simulink model "sgMdl_IO623_FlexRayLoopback"  (R2024b)
settings: Solver=FixedStepAuto  StartTime=0.0  StopTime=inf  RelTol=1e-3  EnableMultiTasking=on
undefined symbols (not defined in the file): IO623
libraries: speedgoatlib_IO623 x8, speedgoatlib_interrupt x1
Description:
  | IO623 - Loopback Test
settings Model: ModifiedByFormat=Speedgoat  SimulationMode=external  Creator=Speedgoat  LastModifiedBy=Speedgoat
settings SolverCC: ConcurrentTasks=on  AlgebraicLoopSolver=TrustRegion  PositivePriorityOrder=on  AutoInsertRateTranBlk=on
settings DataIOCC: SaveFormat=StructureWithTime
settings OptimizationCC: BlockReduction=off  OptimizeBlockIOStorage=off  ReuseModelBlockBuffer=off
settings DebuggingCC: TasksWithSamePriorityMsg=none  UnconnectedInputMsg=warning  UnconnectedOutputMsg=warning  UnconnectedLineMsg=warning
settings HardwareCC: ProdBitPerLong=64  ProdLongLongMode=on  ProdHWDeviceType=Intel->x86-64 (Linux 64)
settings ModelReferenceCC: EnableRefExpFcnMdlSchedulingChecks=on
settings RTWCC: Description=Speedgoat Real-Time Target Machine  SystemTargetFile=speedgoat.tlc  TemplateMakefile=slrealtime_default_tmf  PostCodeGenCommand=sg.model.build.makeCfg(bdroot, buildInfo);  Toolchain=Simulink Real-Time Toolchain  BuildConfiguration=Faster Runs  TargetLang=C++  GPUComputeCapability=3.5  DLArmComputeVersion=19.05
settings SimulinkRealTimeTargetCC: SubcomponentCodeInterfacePackaging=Reusable function  InstructionSetFMA=off  LogToMDFFile=off  SLRTFileLogMaxRuns=10  UseGCCFastMath=on
settings ConfigComp: CovBoundaryAbsTol=1.0e-5

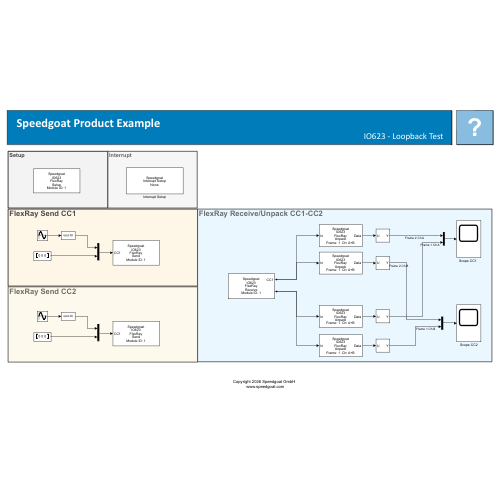
[thumbnail: Simulink's stored preview of the top-level diagram]
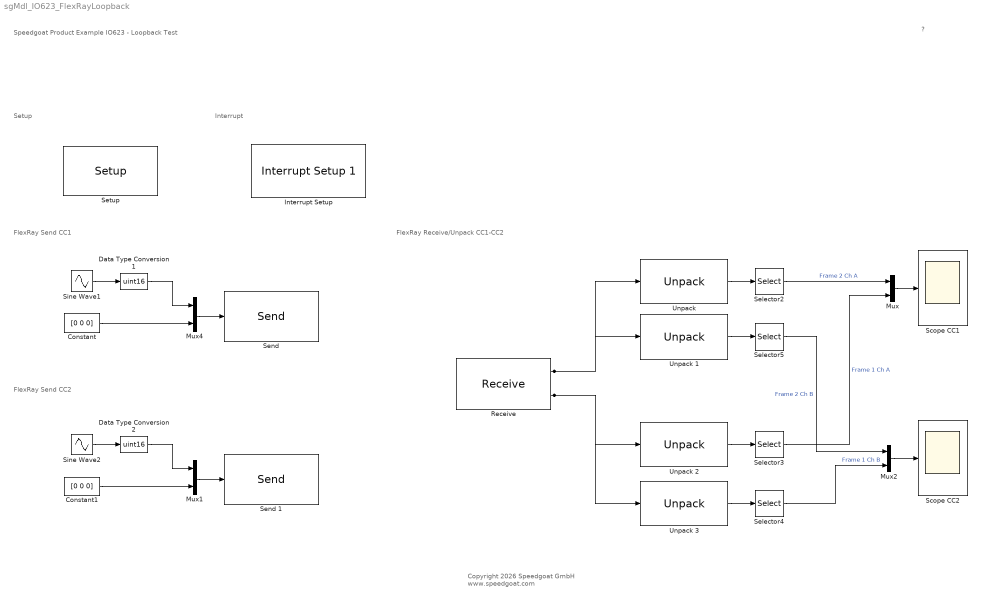
== system sgMdl_IO623_FlexRayLoopback ==
  note: FlexRay Receive/Unpack CC1-CC2
  note: FlexRay Send CC1
  note: FlexRay Send CC2
  note: Interrupt
  note: Setup
  note: Speedgoat Product Example
      | IO623 - Loopback Test
  note: ?
  note: Copyright 2026 Speedgoat GmbH
      |  www.speedgoat.com
  Constant : Constant  Value=[0 0 0]  OutDataTypeStr=uint16
  Constant1 : Constant  Value=[0 0 0]  OutDataTypeStr=uint16
  Data Type Conversion1 : DataTypeConversion  OutDataTypeStr=uint16  SaturateOnIntegerOverflow=off  RndMeth=Floor
  Data Type Conversion2 : DataTypeConversion  OutDataTypeStr=uint16  SaturateOnIntegerOverflow=off  RndMeth=Floor
  Interrupt Setup : speedgoatlib_interrupt/Interrupt Setup 1  parModuleTrigger=on  parPollingMode=off  parPriorityConf=High  parPriority=254  confStartFcn=IO623_start_public  confStopFcn=IO623_stop_public  confIsrFcn=IO623_isr_public  confMapFcn=IO623_map_public  confHookFile=io623_int_hooks.cpp  confIrqNr=-1  confIsPolling=off  confModID=16776961  confSelectedInt=Speedgoat IO623 interrupt  confSelectedId=1  confSelectedChannel=[]  confData=[]  confForcePollingMode=off
  Mux{,1..2,4} (4 alike) : Mux  Inputs=2
  "Receive " : speedgoatlib_IO623/Receive   parModuleId=1  parMaxFrames=10  parSampleTime=-1  parPciSlot=-1  parActiveControllers=[1 1 0 0]
      settings: SourceProductName=Simulink Real-Time: Speedgoat I/O Blockset
  "Scope CC1  " : Scope
  Scope CC2 : Scope
  Selector{2..5} (4 alike) : Selector  InputPortWidth=127  IndexOptions=Index vector (dialog)  Indices=1  OutputSizes=1
  "Send " : speedgoatlib_IO623/Send   parModuleId=1  parCommController=CC1  parSelectionInfo=Frame ID: 1, Channel: A+B, Base: 0, Rep.: 1  parPayloadLength=-1  parSampleTime=-1  parPciSlot=-1  parActiveControllers=[1 1 0 0]
      settings: SourceProductName=Simulink Real-Time: Speedgoat I/O Blockset
  Send 1 : speedgoatlib_IO623/Send   parModuleId=1  parCommController=CC2  parSelectionInfo=Frame ID: 2, Channel: A+B, Base: 0, Rep.: 1  parPayloadLength=-1  parSampleTime=-1  parPciSlot=-1  parActiveControllers=[1 1 0 0]
      settings: SourceProductName=Simulink Real-Time: Speedgoat I/O Blockset
  "Setup " : speedgoatlib_IO623/Setup   parModuleId=1  parPciSlot=-1  parModuleVariant=IO623-2  parChiFile1=config_cc1.chi  parEnableCc1=on  parBusTermination1=on  parChiFile2=config_cc2.chi  parEnableCc2=on  parBusTermination2=off  parEnableCc3=on  parBusTermination3=off  parEnableCc4=on  parBusTermination4=off
      settings: SourceProductName=Simulink Real-Time: Speedgoat I/O Blockset
  Sine Wave1 : Sin  Amplitude=32767  Bias=32768  Frequency=5*2*pi
  Sine Wave2 : Sin  Amplitude=32767  Bias=32768  Frequency=5*2*pi  Phase=2*pi*1/4
  "Unpack " : speedgoatlib_IO623/Unpack   parFrameId=2  parChannels=A  parIgnoreNullFrames=on  parEnPortPayloadPreambleInd=off  parEnPortNullFrameInd=off  parEnPortSyncFrameInd=off  parEnPortStartupFrameInd=off  parEnPortPayloadLength=off  parEnPortHeaderCrc=off  parEnPortCycleCount=off  parEnPortData=on  parEnPortChannel=off  parEnPortValidFrame=off  parEnPortSyntaxError=off  parEnPortContentError=off  parEnPortSlotBoundaryViolation=off  parEnPortTimestamp=off
      settings: SourceProductName=Simulink Real-Time: Speedgoat I/O Blockset
  Unpack 1 : speedgoatlib_IO623/Unpack   parFrameId=2  parChannels=B  parIgnoreNullFrames=on  parEnPortPayloadPreambleInd=off  parEnPortNullFrameInd=off  parEnPortSyncFrameInd=off  parEnPortStartupFrameInd=off  parEnPortPayloadLength=off  parEnPortHeaderCrc=off  parEnPortCycleCount=off  parEnPortData=on  parEnPortChannel=off  parEnPortValidFrame=off  parEnPortSyntaxError=off  parEnPortContentError=off  parEnPortSlotBoundaryViolation=off  parEnPortTimestamp=off
      settings: SourceProductName=Simulink Real-Time: Speedgoat I/O Blockset
  Unpack 2 : speedgoatlib_IO623/Unpack   parFrameId=1  parChannels=A  parIgnoreNullFrames=on  parEnPortPayloadPreambleInd=off  parEnPortNullFrameInd=off  parEnPortSyncFrameInd=off  parEnPortStartupFrameInd=off  parEnPortPayloadLength=off  parEnPortHeaderCrc=off  parEnPortCycleCount=off  parEnPortData=on  parEnPortChannel=off  parEnPortValidFrame=off  parEnPortSyntaxError=off  parEnPortContentError=off  parEnPortSlotBoundaryViolation=off  parEnPortTimestamp=off
      settings: SourceProductName=Simulink Real-Time: Speedgoat I/O Blockset
  Unpack 3 : speedgoatlib_IO623/Unpack   parFrameId=1  parChannels=B  parIgnoreNullFrames=on  parEnPortPayloadPreambleInd=off  parEnPortNullFrameInd=off  parEnPortSyncFrameInd=off  parEnPortStartupFrameInd=off  parEnPortPayloadLength=off  parEnPortHeaderCrc=off  parEnPortCycleCount=off  parEnPortData=on  parEnPortChannel=off  parEnPortValidFrame=off  parEnPortSyntaxError=off  parEnPortContentError=off  parEnPortSlotBoundaryViolation=off  parEnPortTimestamp=off
      settings: SourceProductName=Simulink Real-Time: Speedgoat I/O Blockset
  wires:
  Mux1/1 -> Send 1/1
  Constant1/1 -> Mux1/2
  Selector5/1 -> Mux2/1  "Frame 2 Ch B"
  Selector4/1 -> Mux2/2  "Frame 1 Ch B"
  Sine Wave2/1 -> Data Type Conversion2/1
  "Receive "/1 -> Unpack 1/1, "Unpack "/1
  Data Type Conversion1/1 -> Mux4/1
  Selector3/1 -> Mux/2  "Frame 1 Ch A"
  Mux/1 -> "Scope CC1  "/1
  Data Type Conversion2/1 -> Mux1/1
  Mux2/1 -> Scope CC2/1
  Unpack 2/1 -> Selector3/1
  Unpack 3/1 -> Selector4/1
  "Receive "/2 -> Unpack 2/1, Unpack 3/1
  Selector2/1 -> Mux/1  "Frame 2 Ch A"
  "Unpack "/1 -> Selector2/1
  Sine Wave1/1 -> Data Type Conversion1/1
  Constant/1 -> Mux4/2
  Mux4/1 -> "Send "/1
  Unpack 1/1 -> Selector5/1
